simulink model "GFM_NN_closedloop"  (R2025a)
settings: Solver=FixedStepAuto  StartTime=0.0  StopTime=8  FixedStep=1e-6  RelTol=1e-5
PostLoadFcn:
  | , if any(exist('dsrtsu_mdlpostloadfcn', 'file') == [2, 3, 6]), try dsrtsu_mdlpostloadfcn('Execute', bdroot); catch fprintf('Error in PostLoadFcn (dsrtsu_mdlpostloadfcn) for model "%s":\n %s\n', bdroot, lasterr); end, end,
InitFcn:
  | %% ---------sampling time---------
  | fs=10000;
  | Ts = 1/fs; % 1/fs = sampling period;
  | Tsp=Ts;
  | ws=2*pi*fs;
  | Tc = Ts/1;
  | Tch = inf;
  | % Interrupt shift
  | %Tint=0.25e-6;
  | Tint=0.25e-6;
  | %Tint=0;
  | 
  | %% Frequency
  | fsw = 10e3;
  | Tsp = 1 / fsw;
  | % Ts = 1e-6;
  | 
  | %% Grid parameters
  | Vg_LG_RMS = 110;
  | Vg_LL_RMS = Vg_LG_RMS * sqrt(3);
  | f1 = 50;
  | w1 = f1 * 2 * pi;
  | 
  | Lg = 15e-3;
  | Rg = w1 * Lg * 0.05;
  | 
  | %% GFM converter
  | peak_phase_to_earth = sqrt(2)/sqrt(3);
  | SN_GFM = 4e3;
  | PN_GFM = SN_GFM;
  | Vtr_1 = 132;
  | V_base_GFL = Vtr_1*peak_phase_to_earth;
  | I_base_GFL = SN_GFM*peak_phase_to_earth/Vtr_1;
  | 
  | Vs_LL_RMS = Vg_LL_RMS;
  | VDC = 600;
  | 
  | Ls = 3e-3;
  | Rs = w1 * Ls * 0.05;
  | % Rs = 1e-1;
  | Cf = 10e-6;
  | Rf = 1e-3;
  | % Rf = 1;
  | 
  | %% Base values
  | w_Base = 1;
  | %w_Base = 2*pi*f1;
  | V_Base_GFM = sqrt(2) * Vs_LL_RMS / sqrt(3);      % Peak value
  | S_Base_GFM = SN_GFM;
  | I_Base_GFM = sqrt(2) * (S_Base_GFM / 3) / (V_Base_GFM / sqrt(2));     % Peak value
  | Z_Base_GFM = V_Base_GFM / I_Base_GFM;
  | L_Base_GFM = Z_Base_GFM / w_Base;
  | C_Base_GFM = 1 / (w_Base * Z_Base_GFM);
  | 
  | w1_pu = w1 / w_Base;
  | 
  | %% PU values
  | Ls * w1_pu / Z_Base_GFM
  | Ls_pu = Ls / Z_Base_GFM;
  | Lg_pu = Lg / Z_Base_GFM;
  | ... (+142 lines)
model workspace (MAT data in the model file):
  W1 = [0.530351698399 -0.46726077795 -0.189978018403 0.581505596638 -0.976636350155 0.285457074642 -0.344555467367 -0.823834598064 0.260987460613 -0.174824804068 0.166140690446 -2.19062757492 ... (5120 elements, 64x80)]
  W2 = [0.0236483272165 -0.12587569654 -3.47338819504 -0.292541116476 -0.164569035172 -0.37011295557 -0.0788608714938 -0.34808665514 -0.0821482911706 0.0780714154243 -0.721733689308 -0.485419809818 ... (1024 elements, 16x64)]
  W3 = [-0.129827529192 0.112917125225 -0.211720749736 0.109386667609 -1.40702748299 -1.11484694481 -0.318361610174 0.218052342534 0.374470740557 -0.190498560667 -0.238774597645 0.996348917484 ... (16 elements, 1x16)]
  b1 = [-8.9806804657 -10.8322944641 0.357735663652 -8.11319255829 -12.3089160919 -6.15159845352 -0.239361956716 -10.1425418854 -3.17705559731 -9.53854560852 -2.29398417473 -11.1701593399 ... (64 elements, 64x1)]
  b2 = [-0.136206507683 -0.45766967535 -1.54362010956 -0.556495547295 -0.369174063206 -1.49981951714 -1.85871458054 -0.587826907635 -4.87963867188 -1.14077246189 -0.44449698925 -0.9487388134 ... (16 elements, 16x1)]
  b3 = 2.70423817635
  iqrValues = [999.929682567 999.948806394 999.974126382 1163.68199033 1249.86143465 1016.10909761 999.955656405 999.968539404 999.977085124 999.966554003 999.979581889 999.988183479 ... (80 elements, 1x80)]
  medianValues = [1999.66013382 1999.76293028 1999.73262567 1999.76378275 1999.76361619 1999.77040731 1999.79192245 1999.85691047 1999.87382515 1999.88874694 1999.91524435 1999.91351393 ... (80 elements, 1x80)]
  mu = [-0.108593781339 -0.147308811259 -0.175534555128 -0.136585928467 -0.119784171193 -0.170883245612 -0.185899506459 -0.135931465846 -0.0891217813808 -0.0659545740614 -0.0558679902038 -0.052863332895 ... (80 elements, 1x80)]
  net2 : dlnetwork (value not decoded)
  sigma = [0.7187830922 0.834238393845 0.919900139685 0.688758980318 0.599693957155 0.858339742411 0.965167977116 0.792700626358 0.681503940515 0.658236278259 0.655707879722 0.655775233832 ... (80 elements, 1x80)]
undefined symbols (not defined in the file): DiscIntNeverNeededParam
libraries: spsSeriesRLCBranchLib x18, spsCurrentMeasurementLib x9, simulink x6, spsVoltageMeasurementLib x6, simulink_extras x4, spsGroundLib x4, plecslib_extras x2, deeplib x1, spsDCVoltageSourceLib x1, spsThreePhaseProgrammableVoltageSourceLib x1, spsTwoLevelConverterLib x1, spspowerguiLib x1
(part 3 of 3)

== system GFM_NN_closedloop/Control System/Controller-GFM/GFM_LV/Duty_out/Subsystem10/exp(jwT)1 ==
  dq : Inport
  wt : Inport  Port=2
  Add : Sum  Inputs=+-
  Add1 : Sum
  Demux2 : Demux  Outputs=2
  Mux1 : Mux  Inputs=2
  Product{2..5} (4 alike) : Product  InputSameDT=on  SaturateOnIntegerOverflow=on  OutDataTypeStr=Inherit: Same as first input
  Trigonometric Function : Trigonometry
  Trigonometric Function1 : Trigonometry  Operator=cos
  alphabeta : Outport  VectorParamsAs1DForOutWhenUnconnected=off
  wires:
  wt/1 -> Trigonometric Function/1, Trigonometric Function1/1
  Trigonometric Function/1 -> Product3/2, Product4/2
  Trigonometric Function1/1 -> Product2/2, Product5/2
  Demux2/1 -> Product2/1, Product4/1
  Product3/1 -> Add/2
  Product2/1 -> Add/1
  dq/1 -> Demux2/1
  Add/1 -> Mux1/1
  Add1/1 -> Mux1/2
  Demux2/2 -> Product3/1, Product5/1
  Product5/1 -> Add1/2
  Product4/1 -> Add1/1
  Mux1/1 -> alphabeta/1

== system GFM_NN_closedloop/Control System/Controller-GFM/GFM_LV/PLL/Subsystem7/AlphaBeta -> dq I ==
  alpha : Inport
  beta : Inport  Port=2
  theta : Inport  Port=3
  Fcn2 : Fcn  Expr=cos(u(3))*u(1)+sin(u(3))*u(2)
  Fcn3 : Fcn  Expr=-sin(u(3))*u(1)+cos(u(3))*u(2)
  Mux : Mux  Inputs=3
  d : Outport  VectorParamsAs1DForOutWhenUnconnected=off
  q : Outport  Port=2  VectorParamsAs1DForOutWhenUnconnected=off
  wires:
  beta/1 -> Mux/2
  alpha/1 -> Mux/1
  theta/1 -> Mux/3
  Fcn2/1 -> d/1
  Fcn3/1 -> q/1
  Mux/1 -> Fcn3/1, Fcn2/1

== system GFM_NN_closedloop/Control System/Controller-GFM/GFM_LV/PLL/Subsystem7/Subsystem1 ==
  abc : Inport
  Gain1 : Gain  Gain=2/3  SaturateOnIntegerOverflow=on  OutDataTypeStr=Inherit: Same as input  ParamDataTypeStr=Inherit: Same as input
  Gain3 : Gain  Gain="[ 1   -1/2   -1/2; 0   sqrt(3)/2   -sqrt(3)/2]"  Multiplication=Matrix(K*u) (u vector)  SaturateOnIntegerOverflow=on  OutDataTypeStr=Inherit: Same as input  ParamDataTypeStr=Inherit: Same as input
  alpha_beta : Outport  VectorParamsAs1DForOutWhenUnconnected=off
  wires:
  abc/1 -> Gain3/1
  Gain3/1 -> Gain1/1
  Gain1/1 -> alpha_beta/1

== matlab function GFM_NN_closedloop/Control System/Controller-GFM/GFM_LV/i_transform/MATLAB Function ==
  data: u input; y output; prevVec input
function y = downsample(u, prevVec)
    persistent count;
    if isempty(count)
        count = 0;
    end

    y = prevVec;

    count = count + 1;
    
    if mod(count, 5000) == 0
       y = u;
    end
 

end

== matlab function GFM_NN_closedloop/Control System/Controller-GFM/GFM_LV/PQ_cal/MATLAB Function1 ==
  data: u input; y output
function y = reverse_input(u)
    
    y = flip(u);

== matlab function GFM_NN_closedloop/Control System/Controller-GFM/GFM_LV/PQ_cal/MATLAB Function ==
  data: u input; y output; prevVec input
function y = shiftVector(u, prevVec)
    persistent count last_value;
    if isempty(count)
        count = 0;
        last_value = 0;
    end

    y = prevVec;

    count = count + 1;
    
    if mod(count, 50000) == 0
       last_value = u;
       y = circshift(prevVec, [1, 0]); % Shift right
       y(1) = last_value;
    end

    %y = circshift(prevVec, [1, 0]); % Shift right
    %y(1) = last_value;
   
end
